simulink model "Coherent_BFSK"  (R2013a)
settings: Solver=ode45  StartTime=0.0  StopTime=10/1200  RelTol=1e-3
libraries: commsynccomp2 x1, commrandsrc2 x1
settings Model: Creator=Cedric  LastModifiedBy=Cedric

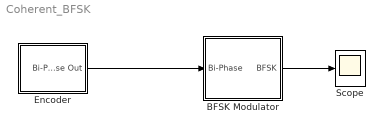
== system Coherent_BFSK ==
  BFSK Modulator : Subsystem
  Encoder : Subsystem
  Scope : Scope
  wires:
  BFSK Modulator/1(BFSK) -> Scope/1
  Encoder/1(Bi-Phase Out) -> BFSK Modulator/1(Bi-Phase)

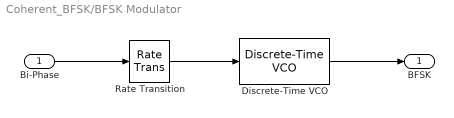
== system Coherent_BFSK/BFSK Modulator ==
  Bi-Phase : Inport
  Discrete-Time VCO : commsynccomp2/Discrete-Time VCO  Ac=5  Fc=1200  Kc=1000  Ph=0  ts=1/(1200*4800)
  Rate Transition : RateTransition  OutPortSampleTime=1/4800
  BFSK : Outport
  wires:
  Discrete-Time VCO/1 -> BFSK/1
  Bi-Phase/1 -> Rate Transition/1
  Rate Transition/1 -> Discrete-Time VCO/1

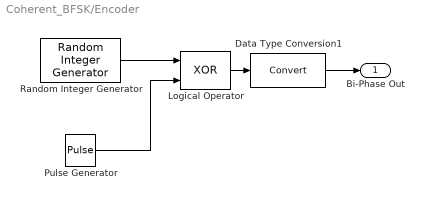
== system Coherent_BFSK/Encoder ==
  Data Type Conversion1 : DataTypeConversion
  Logical Operator : Logic  Operator=XOR  IconShape=distinctive  AllPortsSameDT=off  OutDataTypeStr=boolean
  Pulse Generator : DiscretePulseGenerator  Period=4800  PulseWidth=2400  SampleTime=1/(4800*256)
  Random Integer Generator : commrandsrc2/Random Integer Generator  mul=2  seed=randseed  Ts=1/1200  frameBased=off  sampPerFrame=1  orient=off  outDataType=boolean
  Bi-Phase Out : Outport
  wires:
  Random Integer Generator/1 -> Logical Operator/1
  Logical Operator/1 -> Data Type Conversion1/1
  Pulse Generator/1 -> Logical Operator/2
  Data Type Conversion1/1 -> Bi-Phase Out/1
